simulink model "Fuzzy_Arduion"  (R2019a)
settings: Solver=VariableStepAuto  StartTime=0.0  StopTime=inf  RelTol=1e-3
libraries: instrumentlib x2
settings Model: Creator=Alejoxbg  LastModifiedBy=Alejoxbg

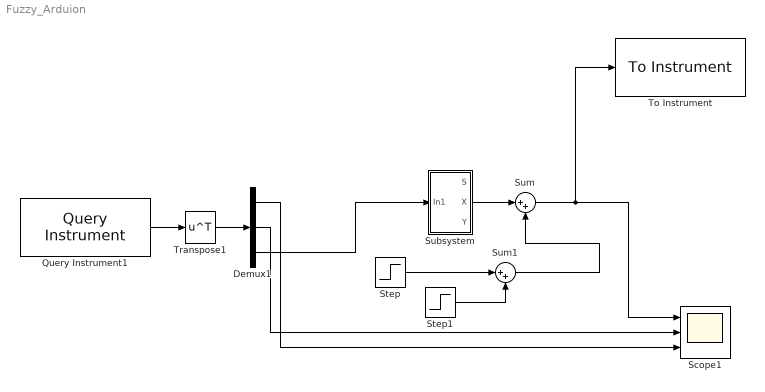
== system Fuzzy_Arduion ==
  Demux1 : Demux  Outputs=3
  Query Instrument1 : instrumentlib/Query Instrument  sampleTime=0.6  isWorkspaceObject=off  timeout=10  inputBufferSize=512  protocol=Serial  serialPort=COM4  baudRate=9600  gpibVendor=Keysight Technologies  boardIndex=0  primaryAddress=1  secondaryAddress=0  visaVendor=Keysight  visaSerialPort=0  chassisIndex=0  logicalAddress=0  tcpRemoteHost='127.0.0.1'  tcpRemotePort=4500  udpRemoteHost='127.0.0.1'  udpRemotePort=9090  visaTCPBoardIndex=0  visaTCPRemoteHost='127.0.0.1'  usbBoardIndex=0  usbManufID=0  usbModelCode=0  usbSerialNumber=0  wsVariableName=s  initAction=None  initCommand='DATA:SOURCE CH1'  initFunction=get  queryCommand='curve?'  responseFormat=ASCII  asciiFormatting='%f;%f;%f'  precision=8-bit integer  byteOrder=Little endian  valuesToRead=1  removeBytes=off  afterOutputAction=Repeat query for new data  enableFrames=on  frameSize=3
      settings: SourceProductName=Instrument Control Toolbox  SourceProductBaseCode=IC
  Scope1 : Scope  NumInputPorts=3
  Step : Step  Time=50  After=0.1  SampleTime=0
  Step1 : Step  Time=100  After=-0.1  SampleTime=0
  Subsystem : Subsystem
  Sum : Sum  Inputs=|++
  Sum1 : Sum  Inputs=|++
  To Instrument : instrumentlib/To Instrument  sampleTime=0.6  isWorkspaceObject=off  timeout=10  inputBufferSize=512  protocol=Serial  serialPort=COM4  baudRate=9600  gpibVendor=ICS Electronics  boardIndex=0  primaryAddress=1  secondaryAddress=0  visaVendor=Keysight  visaSerialPort=0  chassisIndex=0  logicalAddress=0  tcpRemoteHost='127.0.0.1'  tcpRemotePort=4500  udpRemoteHost='127.0.0.1'  udpRemotePort=9090  visaTCPBoardIndex=0  visaTCPRemoteHost='127.0.0.1'  usbBoardIndex=0  usbManufID=0  usbModelCode=0  usbSerialNumber=0  initAction=None  initCommand='4'  initFunction=get  command=''  sendFormat=ASCII  asciiFormatting='%f'  precision=8-bit integer  byteOrder=Little endian
      settings: SourceProductName=Instrument Control Toolbox  SourceProductBaseCode=IC
  Transpose1 : Math  Operator=transpose  SaturateOnIntegerOverflow=on
  wires:
  Demux1/3 -> Subsystem/1(In1)
  Demux1/1 -> Scope1/3
  Transpose1/1 -> Demux1/1
  Query Instrument1/1 -> Transpose1/1
  Demux1/2 -> Scope1/2
  Subsystem/2(X) -> Sum/1
  Sum/1 -> Scope1/1, To Instrument/1
  Step/1 -> Sum1/1
  Step1/1 -> Sum1/2
  Sum1/1 -> Sum/2

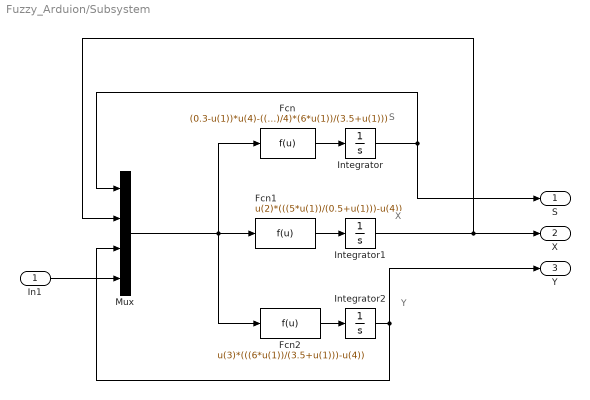
== system Fuzzy_Arduion/Subsystem ==
  note: X
  note: S
  note: Y
  In1 : Inport
  Fcn : Fcn  Expr=(0.3-u(1))*u(4)-((u(2)/4)*(5*u(1))/(0.5+u(1)))-((u(3)/4)*(6*u(1))/(3.5+u(1)))
  Fcn1 : Fcn  Expr=u(2)*(((5*u(1))/(0.5+u(1)))-u(4))
  Fcn2 : Fcn  Expr=u(3)*(((6*u(1))/(3.5+u(1)))-u(4))
  Integrator : Integrator
  Integrator1 : Integrator  InitialCondition=0.1
  Integrator2 : Integrator
  Mux : Mux
  S : Outport
  X : Outport  Port=2
  Y : Outport  Port=3
  wires:
  Fcn/1 -> Integrator/1
  Mux/1 -> Fcn/1, Fcn1/1, Fcn2/1
  Fcn2/1 -> Integrator2/1
  Integrator1/1 -> X/1, Mux/2
  Integrator2/1 -> Y/1, Mux/3
  Integrator/1 -> S/1, Mux/1
  In1/1 -> Mux/4
  Fcn1/1 -> Integrator1/1
